simulink model "compliance"  (R2021b)
settings: Solver=VariableStepAuto  StartTime=0.0  StopTime=5  RelTol=1e-3
undefined symbols (not defined in the file): K, Kd, Kp, xd, xr
settings Model: Creator=fabio  LastModifiedBy=buse

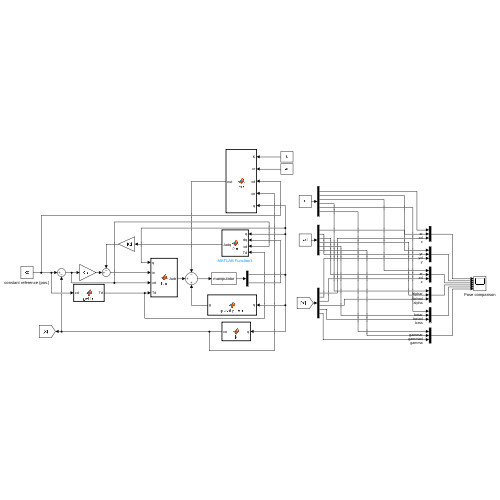
[thumbnail: Simulink's stored preview of the top-level diagram]
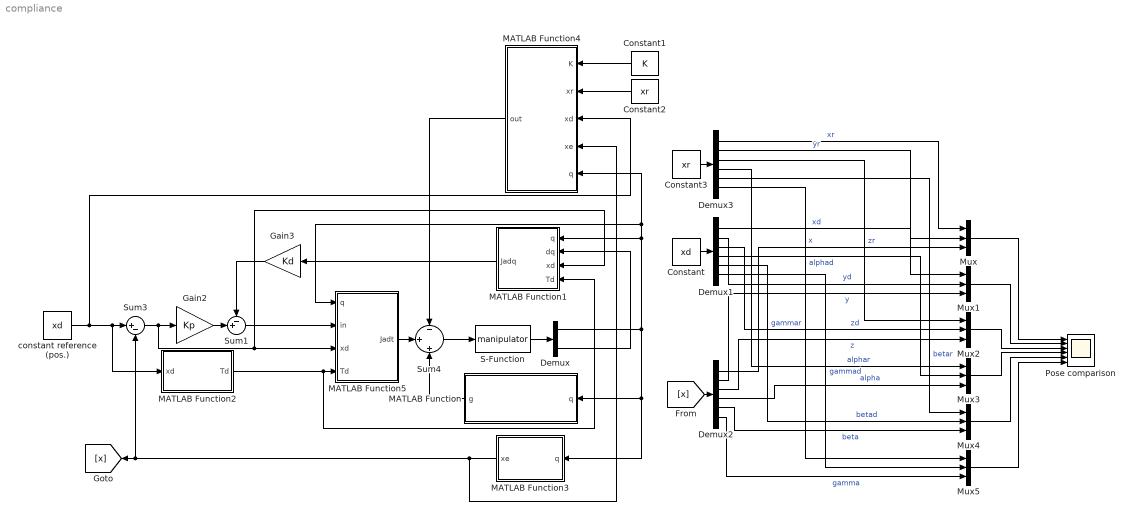
== system compliance ==
  Constant : Constant  Value=xd
  Constant1 : Constant  Value=K
  Constant2 : Constant  Value=xr
  Constant3 : Constant  Value=xr
  Demux : Demux  Outputs=2
  Demux1 : Demux  Outputs=6
  Demux2 : Demux  Outputs=6
  Demux3 : Demux  Outputs=6
  Gain2 : Gain  Gain=Kp
  Gain3 : Gain  Gain=Kd
  MATLAB Function : MATLAB Function  TreatAsAtomicUnit=on
  MATLAB Function1 : MATLAB Function  TreatAsAtomicUnit=on
  MATLAB Function2 : MATLAB Function  TreatAsAtomicUnit=on
  MATLAB Function3 : MATLAB Function  TreatAsAtomicUnit=on
  MATLAB Function4 : MATLAB Function  TreatAsAtomicUnit=on
  MATLAB Function5 : MATLAB Function  TreatAsAtomicUnit=on
  Mux{,1..5} (6 alike) : Mux  Inputs=3
  Pose comparison : Scope  NumInputPorts=6
  S-Function : S-Function  FunctionName=manipulator  Parameters=robot  SFunctionDeploymentMode=off  EnableBusSupport=off
  Sum1 : Sum  Inputs=-+|
  Sum3 : Sum  Inputs=|+-
  Sum4 : Sum  Inputs=-|+|+
  constant reference (pos.) : Constant  Value=xd
  wires:
  Sum3/1 -> MATLAB Function1/3(xd), MATLAB Function5/3(xd), Gain2/1
  Mux1/1 -> Pose comparison/2
  Demux1/4 -> Mux3/2  "alphad"
  Demux1/1 -> Mux/2  "xd"
  Mux4/1 -> Pose comparison/5
  Demux2/1 -> Mux/3  "x"
  Demux1/3 -> Mux2/2  "zd"
  Demux2/4 -> Mux3/3  "alpha"
  Demux1/6 -> Mux5/2  "gammad"
  Gain3/1 -> Sum1/1
  Demux2/2 -> Mux1/3  "y"
  Mux/1 -> Pose comparison/1
  Demux2/3 -> Mux2/3  "z"
  Constant/1 -> Demux1/1
  constant reference (pos.)/1 -> Sum3/1, MATLAB Function2/1(xd), MATLAB Function4/3(xd)
  Mux3/1 -> Pose comparison/4
  Demux2/5 -> Mux4/3  "beta"
  MATLAB Function3/1(xe) -> MATLAB Function4/4(xe), Sum3/2, [x]
  Sum4/1 -> S-Function/1
  Demux1/2 -> Mux1/2  "yd"
  Demux1/5 -> Mux4/2  "betad"
  Mux5/1 -> Pose comparison/6
  MATLAB Function1/1(Jadq) -> Gain3/1
  Mux2/1 -> Pose comparison/3
  Gain2/1 -> Sum1/2
  [x] -> Demux2/1
  S-Function/1 -> Demux/1
  Demux/1 -> MATLAB Function3/1(q), MATLAB Function/1(q), MATLAB Function4/5(q), MATLAB Function5/1(q), MATLAB Function1/1(q)
  Demux2/6 -> Mux5/3  "gamma"
  MATLAB Function5/1(Jadt) -> Sum4/2
  MATLAB Function4/1(out) -> Sum4/1
  Constant1/1 -> MATLAB Function4/1(K)
  Constant2/1 -> MATLAB Function4/2(xr)
  Demux/2 -> MATLAB Function1/2(dq)
  MATLAB Function2/1(Td) -> MATLAB Function1/4(Td), MATLAB Function5/4(Td)
  Sum1/1 -> MATLAB Function5/2(in)
  Constant3/1 -> Demux3/1
  Demux3/1 -> Mux/1  "xr"
  Demux3/2 -> Mux1/1  "yr"
  Demux3/3 -> Mux2/1  "zr"
  Demux3/4 -> Mux3/1  "alphar"
  Demux3/5 -> Mux4/1  "betar"
  Demux3/6 -> Mux5/1  "gammar"
  MATLAB Function/1(g) -> Sum4/3

== matlab function compliance/MATLAB Function1 ==
  data: q input size=3; Jadq output size=6; dq input; xd input; Td input
function Jadq = fcn(q, dq,xd, Td)
    q1 = q(1); q2 = q(2); q3 = q(3);
    % Base to ee transformation matrix
    Te = [-sin(q1)*sin(q3), -cos(q1),  cos(q3)*sin(q1), (2*cos(q1))/5 + (3*sin(q1))/10 + (6*cos(q3)*sin(q1))/25 + q2*sin(q1);
     cos(q1)*sin(q3), -sin(q1), -cos(q1)*cos(q3), (2*sin(q1))/5 - (3*cos(q1))/10 - (6*cos(q1)*cos(q3))/25 - q2*cos(q1);
             cos(q3),        0,          sin(q3),                                                (6*sin(q3))/25 + 3/20;
                   0,        0,                0,                                                                    1];
    % Td frame to ee transformation matrix
    Tde = Td/Te;
    % Euler angles -> rotation matrix  
    s1 = sin(xd(4)); s2 = sin(xd(5)); s3 = sin(xd(6));
    c1 = cos(xd(4)); c2 = cos(xd(5)); c3 = cos(xd(6));
    Rd = [ c1*c3-c2*s1*s3, -c1*s3-c2*c3*s1, s1*s2;
           c3*s1+c1*c2*s3, c1*c2*c3-s1*s3, -c1*s2;
           s2*s3, c3*s2, c2
        ];
    % Rotation matrix -> Euler angles
    R = Tde(1:3,1:3);
    alpha = atan2(R(1,3),R(2,3));
    % pinv(Ta(Phi))
    Ta = [
        [1, 0, 0, 0,       0, 0]
        [0, 1, 0, 0,       0, 0]
        [0, 0, 1, 0,       0, 0]
        [0, 0, 0, 0,       0, 1]  
        [0, 0, 0, cos(alpha), sin(alpha), 0]
        [0, 0, 0, 0, 0, 0]
    ];
    J = [
[(3*cos(q1))/10 - (2*sin(q1))/5 + (6*cos(q1)*cos(q3))/25 + q2*cos(q1),  sin(q1), -(6*sin(q1)*sin(q3))/25]
[(2*cos(q1))/5 + (3*sin(q1))/10 + (6*cos(q3)*sin(q1))/25 + q2*sin(q1), -cos(q1),  (6*cos(q1)*sin(q3))/25]
[                                                                   0,        0,          (6*cos(q3))/25]
[                                                                   0,        0,                -cos(q1)]
[                                                                   0,        0,                -sin(q1)]
[                                                                   1,        0,                       0]
    ];
    % R matrix slide 14 
    R = [Rd' zeros(3,3)
        zeros(3,3) Rd'];
    Jadq = (Ta*R*J)*dq;

== matlab function compliance/MATLAB Function ==
  data: q input; g output
function g = gravityTerm(q)  
    g = getG(q);
end

== matlab function compliance/MATLAB Function2 ==
  data: xd input; Td output
function Td = getTd(xd)
    % Euler angles -> rotation matrix  
    s1 = sin(xd(4)); s2 = sin(xd(5)); s3 = sin(xd(6));
    c1 = cos(xd(4)); c2 = cos(xd(5)); c3 = cos(xd(6));
    Rd = [ c1*c3-c2*s1*s3, -c1*s3-c2*c3*s1, s1*s2;
           c3*s1+c1*c2*s3, c1*c2*c3-s1*s3, -c1*s2;
           s2*s3, c3*s2, c2
        ];
    % Extract the translation vector
    t = xd(1:3);
    Td = [Rd t
        zeros(1,3) 1];

== matlab function compliance/MATLAB Function3 ==
  data: q input size=3; xe output size=6
function xe = k(q)
    q1 = q(1); q2 = q(2); q3 = q(3);
    % Direct kinematics
    xe = [(2*cos(q1))/5 + (3*sin(q1))/10 + (6*cos(q3)*sin(q1))/25 + q2*sin(q1);
         (2*sin(q1))/5 - (3*cos(q1))/10 - (6*cos(q1)*cos(q3))/25 - q2*cos(q1);
         (6*sin(q3))/25 + 3/20;
         q1;
         pi/2 - q3;
         pi/2];

== matlab function compliance/MATLAB Function4 ==
  data: K input; out output size=3; xr input; xd input; xe input; q input
function out = he(K, xr, xd, xe, q)
    q1 = q(1); q2 = q(2); q3 = q(3);
    he = zeros(6,1);
    if xe(2) > xr(2) % Only along y, i.e. only when moving only joint 2
        % In contact
        dxrd = xd-xr;
        dxed = xd-xe;
        dxre = dxrd-dxed;
        he = K*dxre;
    end
    JA = [(3*cos(q1))/10 - (2*sin(q1))/5 + (6*cos(q1)*cos(q3))/25 + q2*cos(q1),  sin(q1), -(6*sin(q1)*sin(q3))/25;
            (2*cos(q1))/5 + (3*sin(q1))/10 + (6*cos(q3)*sin(q1))/25 + q2*sin(q1), -cos(q1),  (6*cos(q1)*sin(q3))/25;
            0,        0,          (6*cos(q3))/25;
            1,        0,                       0;
            0,        0,                      -1;
            0,        0,                       0];
    % Equilibrium point
    out = JA.'*he;

== matlab function compliance/MATLAB Function5 ==
  data: q input size=3; in input; Jadt output size=3; xd input; Td input
function Jadt = fcn(q,in, xd, Td)
    q1 = q(1); q2 = q(2); q3 = q(3);
    % Base to ee transformation matrix
    Te = [-sin(q1)*sin(q3), -cos(q1),  cos(q3)*sin(q1), (2*cos(q1))/5 + (3*sin(q1))/10 + (6*cos(q3)*sin(q1))/25 + q2*sin(q1);
     cos(q1)*sin(q3), -sin(q1), -cos(q1)*cos(q3), (2*sin(q1))/5 - (3*cos(q1))/10 - (6*cos(q1)*cos(q3))/25 - q2*cos(q1);
             cos(q3),        0,          sin(q3),                                                (6*sin(q3))/25 + 3/20;
                   0,        0,                0,                                                                    1];
    % Td frame to ee transformation matrix
    Tde = Td/Te;
    % Rotation matrix -> Euler angles
    R = Tde(1:3,1:3);
    alpha = atan2(R(1,3),R(2,3));
    % pinv(Ta(Phi))
    Ta = [
        [1, 0, 0, 0,       0, 0]
        [0, 1, 0, 0,       0, 0]
        [0, 0, 1, 0,       0, 0]
        [0, 0, 0, 0,       0, 1]  
        [0, 0, 0, cos(alpha), sin(alpha), 0]
        [0, 0, 0, 0, 0, 0]
    ];
    J = [
[(3*cos(q1))/10 - (2*sin(q1))/5 + (6*cos(q1)*cos(q3))/25 + q2*cos(q1),  sin(q1), -(6*sin(q1)*sin(q3))/25]
[(2*cos(q1))/5 + (3*sin(q1))/10 + (6*cos(q3)*sin(q1))/25 + q2*sin(q1), -cos(q1),  (6*cos(q1)*sin(q3))/25]
[                                                                   0,        0,          (6*cos(q3))/25]
[                                                                   0,        0,                -cos(q1)]
[                                                                   0,        0,                -sin(q1)]
[                                                                   1,        0,                       0]
    ];
    % Euler angles -> rotation matrix  
    s1 = sin(xd(4)); s2 = sin(xd(5)); s3 = sin(xd(6));
    c1 = cos(xd(4)); c2 = cos(xd(5)); c3 = cos(xd(6));
    Rd = [ c1*c3-c2*s1*s3, -c1*s3-c2*c3*s1, s1*s2;
           c3*s1+c1*c2*s3, c1*c2*c3-s1*s3, -c1*s2;
           s2*s3, c3*s2, c2
        ];
    % R matrix slide 14 
    R = [Rd' zeros(3,3)
        zeros(3,3) Rd'];
    Jadt = (Ta*R*J)'*in;
